simulink model "Q20"  (Simulink 9.1)
settings: Solver=VariableStepAuto  StartTime=0.0  StopTime=500  RelTol=1e-3
libraries: simulink x1
settings Model: Creator=GamePC  LastModifiedBy=GamePC
settings DataIOCC: SaveFormat=Dataset
settings OptimizationCC: LifeSpan=auto
settings DebuggingCC: UnderspecifiedInitializationDetection=Simplified  MergeDetectMultiDrivingBlocksExec=error  SFUnexpectedBacktrackingDiag=error  SFNoUnconditionalDefaultTransitionDiag=error  SFExecutionAtInitializationDiag=warning
settings HardwareCC: ProdBitPerPointer=64  ProdBitPerSizeT=64  ProdBitPerPtrDiffT=64  ProdLargestAtomicFloat=Float  ProdIntDivRoundTo=Zero  ProdEndianess=LittleEndian  ProdWordSize=64  ProdHWDeviceType=Intel->x86-64 (Windows64)
settings ModelReferenceCC: PropagateSignalLabelsOutOfModel=on
settings CodeAppCC: StateflowObjectComments=off
settings GRTTargetCC: TargetLangStandard=C99 (ISO)  CombineOutputUpdateFcns=on  GRTInterface=off
settings ConfigComp: CovMetricSettings=dwe  CovHtmlReporting=off  CovSaveCumulativeToWorkspaceVar=off  CovSaveSingleToWorkspaceVar=off  CovExternalEMLEnable=on

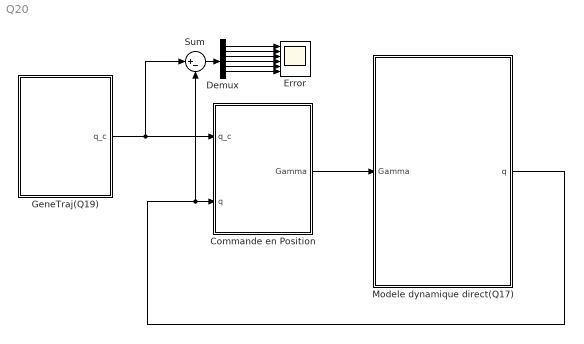
== system Q20 ==
  Commande en Position : Subsystem
  Demux : Demux  Outputs=6
  Error : Scope  NumInputPorts=6
  GeneTraj(Q19) : Subsystem
  Modele dynamique direct(Q17) : Subsystem
  Sum : Sum  Inputs=|+-
  wires:
  Commande en Position/1(Gamma) -> Modele dynamique direct(Q17)/1(Gamma)
  Demux/3 -> Error/3
  Demux/4 -> Error/4
  Demux/1 -> Error/1
  Demux/5 -> Error/5
  Demux/6 -> Error/6
  Sum/1 -> Demux/1
  Modele dynamique direct(Q17)/1(q) -> Sum/2, Commande en Position/2(q)
  GeneTraj(Q19)/1(q_c) -> Sum/1, Commande en Position/1(q_c)
  Demux/2 -> Error/2

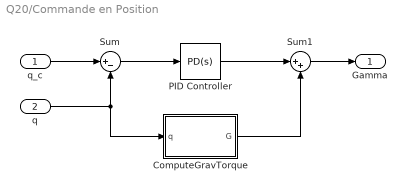
== system Q20/Commande en Position ==
  q_c : Inport
  q : Inport  Port=2
  ComputeGravTorque : MATLAB Function  TreatAsAtomicUnit=on
  PID Controller : simulink/Continuous/PID Controller  Controller=PD  TimeDomain=Continuous-time  SampleTime=-1  IntegratorMethod=Forward Euler  FilterMethod=Forward Euler  Form=Parallel  UseFilter=on  ControllerParametersSource=internal  P=2  I=0  D=0.5  N=100  InitialConditionSource=internal  InitialConditionForIntegrator=0  InitialConditionForFilter=0  ExternalReset=none  LimitOutput=off  UpperSaturationLimit=inf  LowerSaturationLimit=-inf  LinearizeAsGain=on  AntiWindupMode=none  Kb=1  TrackingMode=off  Kt=1  PParamMin=[]  PParamMax=[]  IParamMin=[]  IParamMax=[]  DParamMin=[]  DParamMax=[]  NParamMin=[]  NParamMax=[]  KbParamMin=[]  KbParamMax=[]  KtParamMin=[]  KtParamMax=[]  POutMin=[]  POutMax=[]  IOutMin=[]  IOutMax=[]  DOutMin=[]  DOutMax=[]  NOutMin=[]  NOutMax=[]  KbOutMin=[]  KbOutMax=[]  KtOutMin=[]  KtOutMax=[]  IntegratorOutMin=[]  IntegratorOutMax=[]  FilterOutMin=[]  FilterOutMax=[]  SumOutMin=[]  SumOutMax=[]  SumI1OutMin=[]  SumI1OutMax=[]  SumI2OutMin=[]  SumI2OutMax=[]  SumI3OutMin=[]  SumI3OutMax=[]  SumDOutMin=[]  SumDOutMax=[]  SaturationOutMin=[]  SaturationOutMax=[]  IntegratorContinuousStateAttributes=''  IntegratorStateMustResolveToSignalObject=off  IntegratorRTWStateStorageClass=Auto  FilterContinuousStateAttributes=''  FilterStateMustResolveToSignalObject=off  FilterRTWStateStorageClass=Auto  DifferentiatorICPrevScaledInput=0  DifferentiatorOutMin=[]  DifferentiatorOutMax=[]  FilterDiffOutCoefMin=[]  FilterDiffOutCoefMax=[]  SumDenOutMin=[]  SumDenOutMax=[]  SumNumOutMin=[]  SumNumOutMax=[]  ReciprocalOutMin=[]  ReciprocalOutMax=[]  DivideOutMin=[]  DivideOutMax=[]  TunerSelectOption=Transfer Function Based (PID Tuner App)
  Sum : Sum  Inputs=|+-
  Sum1 : Sum  Inputs=|++
  Gamma : Outport
  wires:
  Sum/1 -> PID Controller/1
  ComputeGravTorque/1(G) -> Sum1/2
  Sum1/1 -> Gamma/1
  PID Controller/1 -> Sum1/1
  q/1 -> ComputeGravTorque/1(q), Sum/2
  q_c/1 -> Sum/1

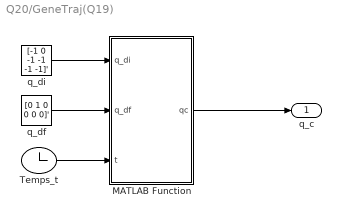
== system Q20/GeneTraj(Q19) ==
  MATLAB Function : MATLAB Function  TreatAsAtomicUnit=on
  "Temps_t " : Clock
  "q_df " : Constant  Value=[0 1 0 0 0 0]'  VectorParams1D=off
  q_di : Constant  Value=[-1 0 -1 -1 -1 -1]'  VectorParams1D=off
  q_c : Outport
  wires:
  MATLAB Function/1(qc) -> q_c/1
  q_di/1 -> MATLAB Function/1(q_di)
  "Temps_t "/1 -> MATLAB Function/3(t)
  "q_df "/1 -> MATLAB Function/2(q_df)

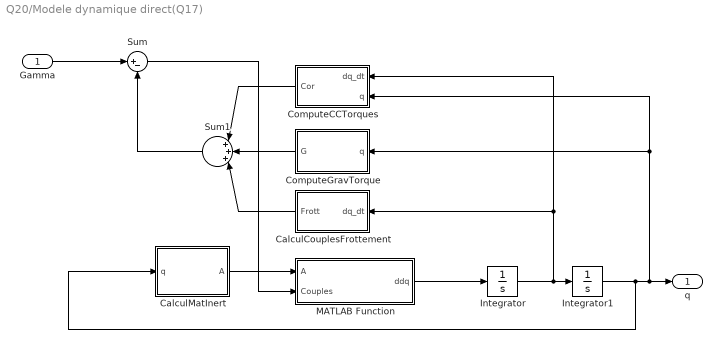
== system Q20/Modele dynamique direct(Q17) ==
  Gamma : Inport
  CalculCouplesFrottement : MATLAB Function  TreatAsAtomicUnit=on
  CalculMatInert : MATLAB Function  TreatAsAtomicUnit=on
  ComputeCCTorques : MATLAB Function  TreatAsAtomicUnit=on
  ComputeGravTorque : MATLAB Function  TreatAsAtomicUnit=on
  Integrator : Integrator
  Integrator1 : Integrator
  MATLAB Function : MATLAB Function  TreatAsAtomicUnit=on
  Sum : Sum  Inputs=|+-
  Sum1 : Sum  Inputs=|+++|
  q : Outport
  wires:
  Gamma/1 -> Sum/1
  Sum1/1 -> Sum/2
  Sum/1 -> MATLAB Function/2(Couples)
  ComputeGravTorque/1(G) -> Sum1/2
  ComputeCCTorques/1(Cor) -> Sum1/1
  Integrator/1 -> ComputeCCTorques/1(dq_dt), CalculCouplesFrottement/1(dq_dt), Integrator1/1
  CalculCouplesFrottement/1(Frott) -> Sum1/3
  Integrator1/1 -> q/1, ComputeCCTorques/2(q), ComputeGravTorque/1(q), CalculMatInert/1(q)
  MATLAB Function/1(ddq) -> Integrator/1
  CalculMatInert/1(A) -> MATLAB Function/1(A)

== matlab function GeneTraj(Q19)/MATLAB Function ==
  data: q_di input double; qc output double; q_df input double; t input double
function qc = GeneTraj(q_di, q_df, t)
    
    tf = 500; % ms     
    D = (q_df - q_di);    
    r = 10 * (t/tf)^3 - 15 * (t/tf)^4 + 6 * (t/tf)^5;   
    qc = q_di + r*D;
end

== matlab function Modele dynamique direct(Q17)/CalculMatInert ==
  data: q input double; A output double size=[6,6]
function A = CalculMatInert(q)
    %set parameter
    m = [15,10,1,7,1,0.5];
    x_G1 = 0; y_G1 = 0; z_G1 = -0.25;
    x_G2 = 0.35; y_G2 = 0; z_G2 = 0;
    x_G3 = 0; y_G3 = -0.1; z_G3 = 0;
    x_G4 = 0; y_G4 = 0; z_G4 = 0;
    x_G5 = 0; y_G5 = 0; z_G5 = 0;
    x_G6 = 0; y_G6 = 0; z_G6 = 0;
    x_G=[x_G1 x_G2 x_G3 x_G4 x_G5 x_G6]';
    y_G=[y_G1 y_G2 y_G3 y_G4 y_G5 y_G6]';
    z_G=[z_G1 z_G2 z_G3 z_G4 z_G5 z_G6]';
    
    iI = zeros(3,3,6);
    iI(:,:,1)=[0.80 0 0.05 ; 0 0.80 0 ; 0.05  0  0.10];
    iI(:,:,2)=[0.10  0  0.10; 0  1.50 0 ; 0.10  0  1.50];
    iI(:,:,3)=[0.05 0 0 ; 0 0.01 0 ; 0 0 0.05];
    iI(:,:,4)=[0.50 0 0 ; 0 0.50 0 ; 0 0 0.05];
    iI(:,:,5)=[0.01 0 0 ; 0 0.01 0 ; 0 0 0.01];
    iI(:,:,6)=[0.01 0 0 ; 0 0.01 0 ; 0 0 0.01];
    
    d3 = 0.7; d = [0,0,d3,0,0,0];
    r1 = 0.5; r4 = 0.2; r = [r1,0,0,r4,0,0];   
    alpha = [ 0 , pi/2 , 0 , pi/2 , -pi/2 , pi/2 ];
    theta = zeros(6,1);
    theta = [q(1) q(2) q(3)+pi/2 q(4) q(5) q(6)]';
    Rred = [100 100 100 70 70 70];
    Jm = 1e-5*[1 1 1 1 1 1];
    %initialization of result
    %A = zeros(size(q,1),size(q,1));
    A = zeros(6,6);
    
    g_0i = eye(4);
    g_elem = eye(4);
    OJv_Gi = zeros(3,6);
    OJ_wi = zeros(3,6);
    [OJv_Gi,OJ_wi] = CalculMatriceJacobienneGi(alpha, d, theta, r, x_G, y_G, z_G);
    
    for i = 1:length(q)
        OPreproduitVect_OiGi = [0, -z_G(i), y_G(i);z_G(i),0,-x_G(i);-y_G(i),x_G(i),0];
        %mH = m(i)*OPreproduitVect_OiGi*OPreproduitVect_OiGi
        iI_Gi = iI(:,:,i)+m(i)*OPreproduitVect_OiGi*OPreproduitVect_OiGi;
        
        g_elem = TransformMatElem(alpha(i),d(i),theta(i),r(i));
        g_0i = g_0i*g_elem;
        ROi = g_0i(1:3,1:3);
        
        %OI_Gi = ROi(:,:,i)*iI_Gi*ROi(:,:,i)';
        OI_Gi = ROi*iI_Gi*ROi';
        A = A + (m(i)*OJv_Gi(:,:,i)')*OJv_Gi(:,:,i)+(OJ_wi(:,:,i)')*OI_Gi*OJ_wi(:,:,i);       
    end
A = A + diag(Rred.^2.*Jm);
end

== matlab function Modele dynamique direct(Q17)/ComputeCCTorques ==
  data: dq_dt input double; q input double; Cor output double size=[6,1]
function Cor = fcn(dq_dt, q)
    Cor = zeros(6,1);
    Cor =ComputeCCTorques(q,dq_dt)'; 

end

== matlab function Modele dynamique direct(Q17)/MATLAB Function ==
  data: A input double size=[6,6]; ddq output double size=6; Couples input double size=[6,1]
function ddq = fcn(A, Couples)

ddq = A\Couples;
end

== matlab function Modele dynamique direct(Q17)/ComputeGravTorque ==
  data: q input double; G output double size=6
function G = fcn(q)
    
    G = ComputeGravTorque(q);

end

== matlab function Modele dynamique direct(Q17)/CalculCouplesFrottement ==
  data: dq_dt input double; Frott output double size=6
function Frott = fcn(dq_dt)
    %parametres
    Fv = 10*ones(6,1);
    
    %Fonction donnée à l'interieure du TP
    Frott = diag(dq_dt)*Fv;
   
end

== matlab function Commande en Position/ComputeGravTorque ==
  data: q input double; G output double size=6
function G = fcn(q)
    
    G = ComputeGravTorque(q);

end
